simulink model "sim"  (R2025a)
settings: Solver=VariableStepAuto  StartTime=0.0  StopTime=0.1  RelTol=1e-3
values from neighbouring files (symbols this model uses):
  J_sum = 35.9e-7    (= 3.59e-06)    [lw5.m]
  k_m = 19.9e-3    (= 0.0199)    [lw5.m]
  L_a = 0.070e-3    (= 7e-05)    [lw5.m]
  R_a = 0.358    [lw5.m]
  U_nom = 18    [lw5.m]
  w_0 = n_0 * 2 * pi / 60    (= 889.070720966)    [lw5.m]
libraries: simulink x3
settings Model: Creator=user  LastModifiedBy=user

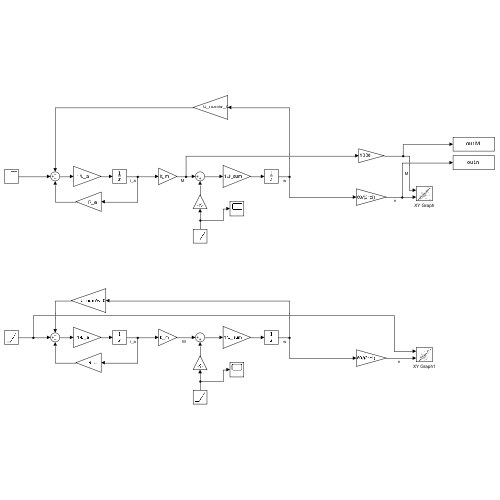
[thumbnail: Simulink's stored preview of the top-level diagram]
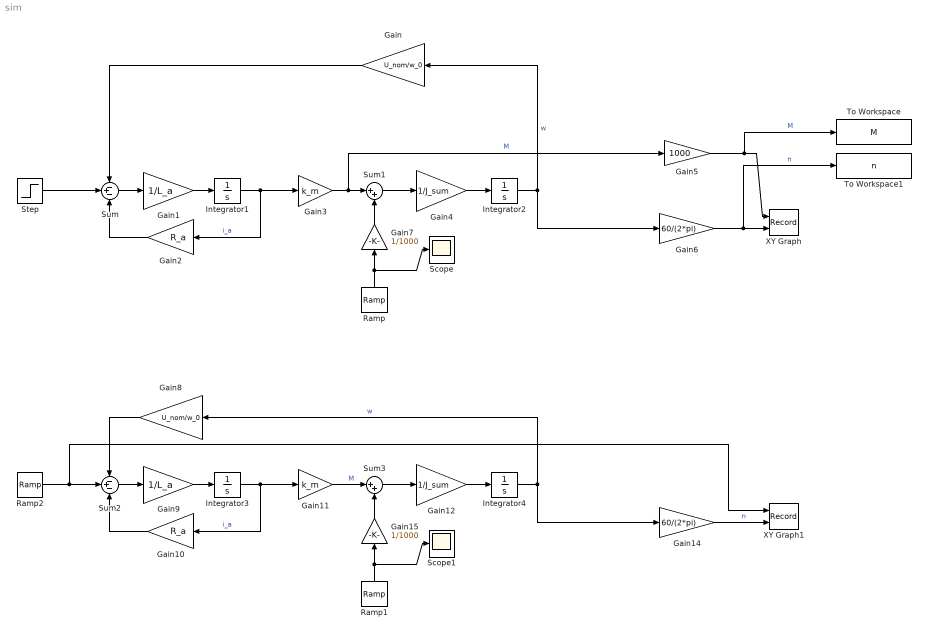
== system sim ==
  Gain : Gain  Gain=U_nom/w_0
  Gain1 : Gain  Gain=1/L_a
  Gain10 : Gain  Gain=R_a
  Gain11 : Gain  Gain=k_m
  Gain12 : Gain  Gain=1/J_sum
  Gain14 : Gain  Gain=60/(2*pi)
  Gain15 : Gain  Gain=1/1000
  Gain2 : Gain  Gain=R_a
  Gain3 : Gain  Gain=k_m
  Gain4 : Gain  Gain=1/J_sum
  Gain5 : Gain  Gain=1000
  Gain6 : Gain  Gain=60/(2*pi)
  Gain7 : Gain  Gain=1/1000
  Gain8 : Gain  Gain=U_nom/w_0
  Gain9 : Gain  Gain=1/L_a
  Integrator{1..4} (4 alike) : Integrator
  Ramp : simulink/Sources/Ramp  slope=1/60  start=0  InitialOutput=1
  Ramp1 : simulink/Sources/Ramp  slope=1/60  start=0  InitialOutput=1
  Ramp2 : simulink/Sources/Ramp  slope=18/0.1  start=0  InitialOutput=0
  Scope : Scope
      settings: ActiveDisplayYMinimum=-1  ActiveDisplayYMaximum=1
  Scope1 : Scope
      settings: ActiveDisplayYMinimum=-1  ActiveDisplayYMaximum=1
  Step : Step  Time=0  After=U_nom  SampleTime=0
  Sum : Sum  Inputs=-+-
  Sum1 : Sum  Inputs=|++
  Sum2 : Sum  Inputs=-+-
  Sum3 : Sum  Inputs=|++
  To Workspace : ToWorkspace  VariableName=M  SaveFormat=Timeseries  SampleTime=-1
  To Workspace1 : ToWorkspace  VariableName=n  SaveFormat=Timeseries  SampleTime=-1
  XY Graph : Record  NumPorts=2.0  FileSettingsInternal="{\"entries\":[{\"content\":{\"excelSettings\":{\"content\":{},\"type\":\"Streamout.ExcelSettings\"},\"parquetSettings\":{\"content\":{},\"type\":\"Streamout.ParquetSettings\"}},\"type\":\"Streamout.FileSettingStorage\",\"uuid\":\"\"}],\"packageUris\":[\"http:\\/\\/schema.mathworks.com\\/mf0\\/streamout_blocks\\/R2020a\"],\"version\":\"1.0\"}"  FrameSettings=[0, 0]  Layout=[1 1]  SignalsInternal="{\"entries\":[{\"content\":{\"signals\":[{\"content\":{\"blockPath\":[],\"dimensions\":[1],\"domain\":\"\",\"lineColor\":\"#a2142f\",\"plots\":[ 1 ],\"port\":1,\"sid\":[\"\"],\"signalID\":1,\"signalName\":\"M\"},\"type\":\"RecordBlkView.Signal\",\"uuid\":\"\"},{\"content\":{\"blockPath\":[],\"dimensions\":[1],\"domain\":\"\",\"lineColor\":\"#139fff\",\"plots\":[ 1 ],\"port\":2,\"sid\":[\"\"],\"signalID\":2,\"signalName\":\"n\"},\"type\":\"RecordBlkView.Signal\",\"uuid\":\"\"}]},\"type\":\"RecordBlkView.InputSignals\",\"uuid\":\"\"}],\"packageUris\":[\"http:\\/\\/schema.mathworks.com\\/mf0\\/streamout_blocks\\/R2020a\"],\"version\":\"1.0\"}"  VisualizationBindings="{\"xyplotplugin\":{\"info\":[{\"series\":[{\"bindingParametersList\":[{\"parameter\":\"X-Axis\",\"signalID\":1,\"signalName\":\"M\"},{\"parameter\":\"Y-Axis\",\"signalID\":2,\"signalName\":\"n\"}],\"seriesID\":0}],\"subplotID\":1}]}}"  CompatibilityTag=XY
  XY Graph1 : Record  NumPorts=2.0  FileSettingsInternal="{\"entries\":[{\"content\":{\"excelSettings\":{\"content\":{},\"type\":\"Streamout.ExcelSettings\"},\"parquetSettings\":{\"content\":{},\"type\":\"Streamout.ParquetSettings\"}},\"type\":\"Streamout.FileSettingStorage\",\"uuid\":\"\"}],\"packageUris\":[\"http:\\/\\/schema.mathworks.com\\/mf0\\/streamout_blocks\\/R2020a\"],\"version\":\"1.0\"}"  FrameSettings=[0, 0]  Layout=[1 1]  SignalsInternal="{\"entries\":[{\"content\":{\"signals\":[{\"content\":{\"blockPath\":[],\"dimensions\":[1],\"domain\":\"\",\"lineColor\":\"#a2142f\",\"plots\":[ 1 ],\"port\":1,\"sid\":[\"\"],\"signalID\":1,\"signalName\":\"Ramp2\"},\"type\":\"RecordBlkView.Signal\",\"uuid\":\"\"},{\"content\":{\"blockPath\":[],\"dimensions\":[1],\"domain\":\"\",\"lineColor\":\"#139fff\",\"plots\":[ 1 ],\"port\":2,\"sid\":[\"\"],\"signalID\":2,\"signalName\":\"n\"},\"type\":\"RecordBlkView.Signal\",\"uuid\":\"\"}]},\"type\":\"RecordBlkView.InputSignals\",\"uuid\":\"\"}],\"packageUris\":[\"http:\\/\\/schema.mathworks.com\\/mf0\\/streamout_blocks\\/R2020a\"],\"version\":\"1.0\"}"  VisualizationBindings="{\"xyplotplugin\":{\"info\":[{\"series\":[{\"bindingParametersList\":[{\"parameter\":\"X-Axis\",\"signalID\":1,\"signalName\":\"Ramp2\"},{\"parameter\":\"Y-Axis\",\"signalID\":2,\"signalName\":\"n\"}],\"seriesID\":0}],\"subplotID\":1}]}}"  CompatibilityTag=XY
  wires:
  Step/1 -> Sum/2
  Sum/1 -> Gain1/1
  Gain1/1 -> Integrator1/1
  Integrator1/1 -> Gain3/1, Gain2/1  "i_a"
  Gain2/1 -> Sum/3
  Gain3/1 -> Gain5/1, Sum1/1  "M"
  Ramp/1 -> Gain7/1, Scope/1
  Sum1/1 -> Gain4/1
  Gain4/1 -> Integrator2/1
  Integrator2/1 -> Gain6/1, Gain/1  "w"
  Gain/1 -> Sum/1
  Gain5/1 -> To Workspace/1, XY Graph/1  "M"
  Gain6/1 -> To Workspace1/1, XY Graph/2  "n"
  Gain7/1 -> Sum1/2
  Gain11/1 -> Sum3/1  "M"
  Gain10/1 -> Sum2/3
  Integrator4/1 -> Gain14/1, Gain8/1  "w"
  Gain12/1 -> Integrator4/1
  Ramp2/1 -> XY Graph1/1, Sum2/2
  Gain8/1 -> Sum2/1
  Sum3/1 -> Gain12/1
  Gain14/1 -> XY Graph1/2  "n"
  Ramp1/1 -> Gain15/1, Scope1/1
  Gain9/1 -> Integrator3/1
  Sum2/1 -> Gain9/1
  Gain15/1 -> Sum3/2
  Integrator3/1 -> Gain11/1, Gain10/1  "i_a"
